simulink model "Motor_speed_control"  (R2020a)
settings: Solver=VariableStepAuto  StartTime=0.0  StopTime=10.0  RelTol=1e-3
values from neighbouring files (symbols this model uses):
  b = 0.1    [Motor_speed_control.sldd]    (also in week3Challenge3_1640261398.mat = 15; week3Challenge3_1_1640261402.mat = 15)
  J = 0.01    [Motor_speed_control.sldd]
  K = 0.01    [Motor_speed_control.sldd]
  L = 1.2    [Motor_speed_control.sldd]
  R = 5.0    [Motor_speed_control.sldd]
libraries: simulink x1
settings Model: DataDictionary=Motor_speed_control.sldd  Creator=NIKITA  LastModifiedBy=NIKITA

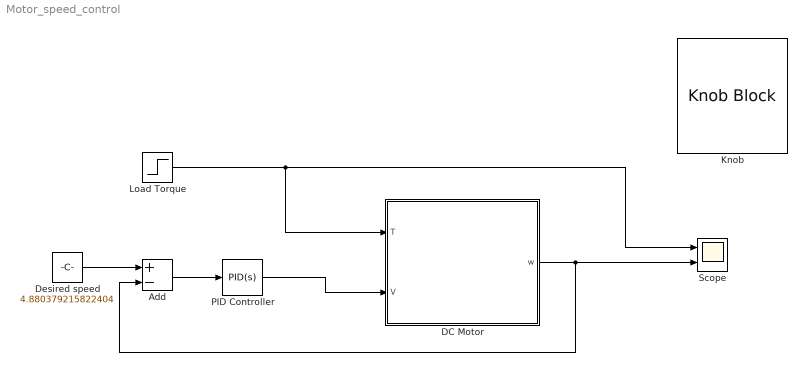
== system Motor_speed_control ==
  Add : Sum  Inputs=+-
  DC Motor : Subsystem
      mask Display: image('Motor1.jpg'); % Use "Edit Image" on toolstrip to change.
  Desired speed : Constant  Value=4.880379215822404
  Knob : KnobBlock  ScaleMax=10
  Load Torque : Step  Time=6  After=3  SampleTime=0
  PID Controller : simulink/Continuous/PID Controller  Controller=PID  Form=Parallel  TimeDomain=Continuous-time  UseExternalTs=off  SampleTime=-1  IntegratorMethod=Forward Euler  FilterMethod=Forward Euler  ControllerParametersSource=internal  P=102.17939753082  I=455.89014489651  D=4.84602769427721  UseFilter=on  N=737.766052005397  TunerSelectOption=Transfer Function Based (PID Tuner App)  InitialConditionSource=internal  InitialConditionForIntegrator=0  InitialConditionForFilter=0  DifferentiatorICPrevScaledInput=0  ExternalReset=none  TrackingMode=off  Kt=1  LimitOutput=off  UpperSaturationLimit=inf  LowerSaturationLimit=-inf  LinearizeAsGain=on  AntiWindupMode=none  Kb=1  POutMin=[]  POutMax=[]  IOutMin=[]  IOutMax=[]  DOutMin=[]  DOutMax=[]  NOutMin=[]  NOutMax=[]  SumOutMin=[]  SumOutMax=[]  SaturationOutMin=[]  SaturationOutMax=[]  PParamMin=[]  PParamMax=[]  IParamMin=[]  IParamMax=[]  DParamMin=[]  DParamMax=[]  NParamMin=[]  NParamMax=[]  KbParamMin=[]  KbParamMax=[]  KtParamMin=[]  KtParamMax=[]  KbOutMin=[]  KbOutMax=[]  KtOutMin=[]  KtOutMax=[]  IntegratorOutMin=[]  IntegratorOutMax=[]  FilterOutMin=[]  FilterOutMax=[]  SumI1OutMin=[]  SumI1OutMax=[]  SumI2OutMin=[]  SumI2OutMax=[]  SumI3OutMin=[]  SumI3OutMax=[]  SumI4OutMin=[]  SumI4OutMax=[]  SumDOutMin=[]  SumDOutMax=[]  DifferentiatorOutMin=[]  DifferentiatorOutMax=[]  FilterDiffOutCoefMin=[]  FilterDiffOutCoefMax=[]  ReciprocalOutMin=[]  ReciprocalOutMax=[]  SumDenOutMin=[]  SumDenOutMax=[]  SumNumOutMin=[]  SumNumOutMax=[]  DivideOutMin=[]  DivideOutMax=[]  UdiffTsProdOutMin=[]  UdiffTsProdOutMax=[]  NTsProdOutMin=[]  NTsProdOutMax=[]  UintegralTsProdOutMin=[]  UintegralTsProdOutMax=[]  UngainTsProdOutMin=[]  UngainTsProdOutMax=[]  IntegratorContinuousStateAttributes=''  IntegratorStateMustResolveToSignalObject=off  IntegratorRTWStateStorageClass=Auto  FilterContinuousStateAttributes=''  FilterStateMustResolveToSignalObject=off  FilterRTWStateStorageClass=Auto  ParallelPVariant=InternalParameters  IdealPVariant=Disabled  IVariant=InternalParameters  DVariant=InternalParameters  IntegratorVariant=Continuous  SatVariant=Disabled  AWVariant=Passthrough  PCopyVariant=Disabled  TRVariant=Disabled  FdbkBlocksVariant=Forward  IdealPFdbkVariant=Disabled  SatFdbkVariant=Disabled  DerivativeFilterVariant=ContFilter  NVariant=InternalParameters  NCopyVariant=Disabled  FilterICVariant=InternalICsFilter  IntegratorICVariant=InternalICs  ExternalResetVariant=Disabled  TRSumVariant=Passthrough  SumFdbkVariant=Disabled  SumVariant=Sum_PID  TsampFilterVariant=InternalTs  TsampNgainVariant=Passthrough  TsampIntegralVariant=Passthrough
  Scope : Scope  NumInputPorts=2
  wires:
  Load Torque/1 -> Scope/1, DC Motor/1(T)
  DC Motor/1(w) -> Scope/2, Add/2
  Add/1 -> PID Controller/1
  PID Controller/1 -> DC Motor/2(V)
  Desired speed/1 -> Add/1

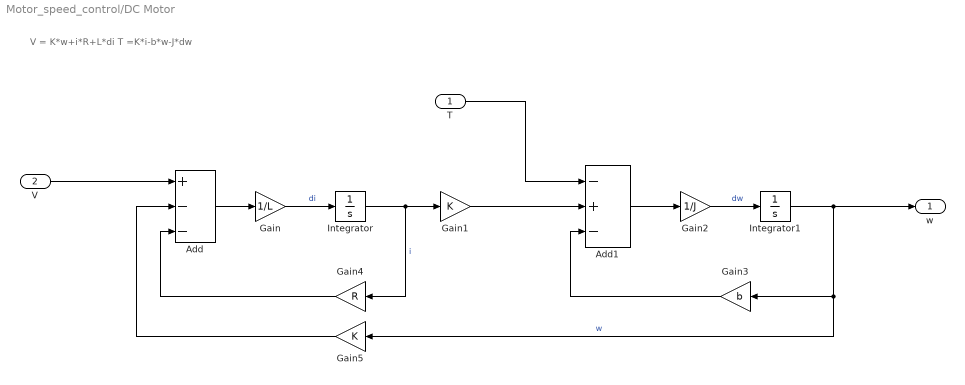
== system Motor_speed_control/DC Motor ==
  note: V = K*w+i*R+L*di
      | T =K*i-b*w-J*dw
  T : Inport
  V : Inport  Port=2
  Add : Sum  Inputs=+--
  Add1 : Sum  Inputs=-+-
  Gain : Gain  Gain=1/L
  Gain1 : Gain  Gain=K
  Gain2 : Gain  Gain=1/J
  Gain3 : Gain  Gain=b
  Gain4 : Gain  Gain=R
  Gain5 : Gain  Gain=K
  Integrator : Integrator
  Integrator1 : Integrator
  w : Outport
  wires:
  Add1/1 -> Gain2/1
  Integrator1/1 -> w/1, Gain5/1, Gain3/1  "w"
  Integrator/1 -> Gain4/1, Gain1/1  "i"
  Gain4/1 -> Add/3
  Gain/1 -> Integrator/1  "di"
  Add/1 -> Gain/1
  T/1 -> Add1/1
  Gain3/1 -> Add1/3
  Gain1/1 -> Add1/2
  Gain5/1 -> Add/2
  Gain2/1 -> Integrator1/1  "dw"
  V/1 -> Add/1
